simulink model "GPC"  (R2025b)
settings: Solver=FixedStepAuto  StartTime=0.0  StopTime=10.0  RelTol=1e-3
model workspace (MAT data in the model file):
  A = reshape([1 1 1 1 1 1 1 1 1 0.0375840959276 -0.0138679170576 -0.26090854365 0.179130502621 0.033894052833 0.0236937396522 0.00188563424393 -0.0137292088517 -0.225147986097 -0.282059074714 -0.0208812255081 0.110151665356 0.251260446677 -0.117899657826 -0.166134716199 -0.197559283491 -0.0255196194892 -0.044091775752 -0.336519979766 0.0187297142758 0.0478749224565 -0.137698933084 -0.35438494619 0.192962428222 0.00475946983706 0.0213883941121 -0.31920636287 -0.0980246146855 0.0103154407684 -0.0398902297506 0.0254465336583 -0.176213728897 -0.0657108585119 -0.0426588905364 0.00598757531626 -0.0347101416777 -0.0960427281846 0.0145828177398 -0.0190829804402 0.0914615693001 -0.160320038871 -0.147671747218 0.0154294464386 0.00151624371842 -0.102514250384], [3 3 6])
  B = reshape([0.00459780777595 1.42712475674e-05 -0.000408041445028 -0.00237157306223 0.00119304873837 0.000482775458328 0.00223132451004 0.000286686912328 0.00599135916028 0.0148665205586 5.139693558e-05 -0.00265500051912 -0.00735163394133 0.00391460700889 0.00243583441326 0.00755730776847 0.000748730221682 0.0148040671963 0.00740132665718 -0.000229008808218 -0.00369283887868 -0.00297542223091 0.00220653401484 0.00209157033751 0.00350399653917 -9.59277212105e-05 0.0030543274579 0.00490088499125 -0.000268745976113 -0.000437929455165 -0.00192593035877 0.00199079743513 0.000615437038067 0.000339606715612 -0.000260130070202 0.00641986430148 0.00188631931206 -6.20353133168e-05 -0.000608242812709 -0.00124764831245 0.000778872732744 0.00128937420791 0.000541054894972 5.56413892428e-05 0.000905590664489 0.000995289355196 -6.55613468166e-05 -0.000860934223846 -0.0004545573316 0.000285028917598 0.000527317246035 -0.000728392089223 -0.000148880686854 0.00124465963027], [3 3 6])
  N1 = 1
  N2 = 15
  Nu = 1
  alpha = 0.5
  lam = [0.2 0.08 0.5]
values from neighbouring files (symbols this model uses):
  Ts_ctrl = 0.1    [ctrlSys.sldd]
  u_b = 0.5864    [ctrlSys.sldd]
settings Model: DataDictionary=ctrlSys.sldd  Creator=LYG  LastModifiedBy=LYG

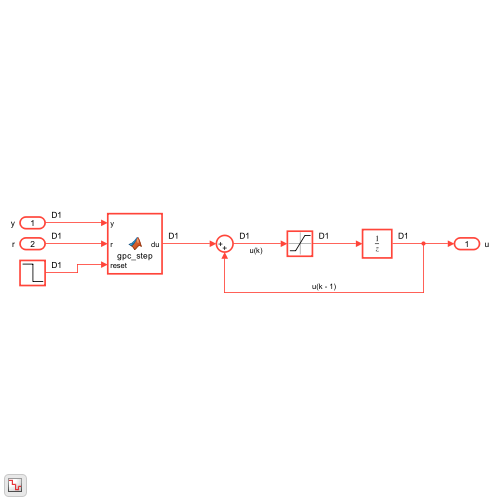
[thumbnail: Simulink's stored preview of the top-level diagram]
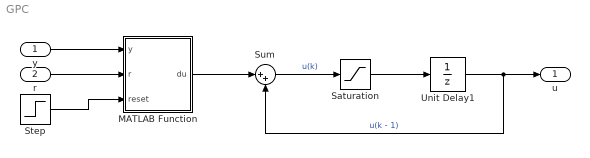
== system GPC ==
  y : Inport
  r : Inport  Port=2
  MATLAB Function : MATLAB Function  TreatAsAtomicUnit=on  SystemSampleTime=Ts_ctrl
  Saturation : Saturate  UpperLimit=1.12  LowerLimit=-1.08
  Step : Step  Time=0.5  Before=1  After=0  SampleTime=Ts_ctrl
  Sum : Sum  Inputs=|++
  Unit Delay1 : UnitDelay  InitialCondition=u_b  SampleTime=-1  HasFrameUpgradeWarning=on
  u : Outport
  wires:
  y/1 -> MATLAB Function/1(y)
  r/1 -> MATLAB Function/2(r)
  Saturation/1 -> Unit Delay1/1
  Sum/1 -> Saturation/1  "u(k)"
  MATLAB Function/1(du) -> Sum/1
  Unit Delay1/1 -> u/1, Sum/2  "u(k - 1)"
  Step/1 -> MATLAB Function/3(reset)

== matlab function GPC/MATLAB Function ==
  data: y input size=[3 1]; du output size=[3 1]; r input size=[3 1]; A parameter; B parameter; N1 parameter size=[1 1]; N2 parameter size=[1 1]; Nu parameter size=[1 1]; alpha parameter size=[1 1]; lam parameter size=[1 3]; reset input size=[1 1]
function du = gpc_step(y, r, A, B, N1, N2, Nu, alpha, lam, reset)
%GPC_STEP  One-step 3x3 GPC move for a CARIMA/ARIMA model with incremental control.
%   Codegen-friendly version for MATLAB Function blocks (no cell arrays).
%
%   A and B must be numeric arrays sized:
%     A: 3x3x(na+1) with A(:,:,1) == 1
%     B: 3x3x(nb+1)
%
%   Computes free response F and reference trajectory R, then applies
%   ΔU* = (G'G+λI)^{-1} G' (R-F) and outputs Δu(k) for each input.
%   Maintains histories of Δy and Δu between calls for the predictor.
    persistent K y_prev dy_hist du_hist last_A last_B last_N1 last_N2 last_Nu last_lam init_flag

    % Reset handling for MATLAB Function block.
    if isempty(init_flag)
        init_flag = true;
    end
    if reset
        init_flag = true;
        du = zeros(3, 1);
        return;
    end

    % Initialize cached parameters to avoid use-before-assign errors.
    if isempty(last_A)
        last_A = A;
        last_B = B;
        last_N1 = N1;
        last_N2 = N2;
        last_Nu = Nu;
        last_lam = lam;
    end

    % Cache the gain matrix unless model/horizons/weight change.
    if init_flag || isempty(K) || isempty(last_A) || isempty(last_B) || ...
            ~isequal(A, last_A) || ~isequal(B, last_B) || ...
            N1 ~= last_N1 || N2 ~= last_N2 || Nu ~= last_Nu || ~isequal(lam, last_lam)
        G = gmat(A, B, N1, N2, Nu);
        Lam = eye(3 * Nu);
        for i = 1:3
            r0 = (i - 1) * Nu + 1;
            Lam(r0:r0+Nu-1, r0:r0+Nu-1) = lam(i) * Lam(r0:r0+Nu-1, r0:r0+Nu-1);
        end
        K = (G' * G + Lam) \ G';
        last_A = A;
        last_B = B;
        last_N1 = N1;
        last_N2 = N2;
        last_Nu = Nu;
        last_lam = lam;
    end

    y = y(:);
    r = r(:);
    if numel(y) ~= 3 || numel(r) ~= 3
        error('y and r must be 3x1 vectors.');
    end

    if isscalar(alpha)
        alpha_vec = repmat(alpha, 3, 1);
    elseif numel(alpha) == 3
        alpha_vec = alpha(:);
    else
        error('alpha must be a scalar or a 3-element vector.');
    end

    % Initialize state history on first call.
    if init_flag || isempty(y_prev)
        y_prev = y;
    end
    na = size(A, 3) - 1;
    nb = size(B, 3) - 1;
    if init_flag || isempty(dy_hist)
        dy_hist = zeros(3, max(na, 1));
    end
    if init_flag || isempty(du_hist)
        du_hist = zeros(3, nb + 1);
    end
    init_flag = false;

    % Current output increment.
    dy_k = y - y_prev;

    % Build histories that include the current sample for free response.
    if na > 0
        dy_hist_use = [dy_k, dy_hist(:, 1:end-1)];
    else
        dy_hist_use = dy_hist(:, 1:1);
    end
    % Free response assumes Δu(k) = 0 (future moves handled by G*ΔU).
    du_hist_use = [zeros(3, 1), du_hist(:, 1:end-1)];

    % Free response over N1..N2.
    F = fmat(A, B, N1, N2, y, dy_hist_use, du_hist_use);

    % Reference trajectory over N1..N2 with exponential smoothing.
    Rfull = zeros(N2+1, 3);
    Rfull(1, :) = y.';
    for i = 2:N2+1
        alpha_row = alpha_vec.';
        Rfull(i, :) = alpha_row .* Rfull(i - 1, :) + (1 - alpha_row) .* r.';
    end
    rows = N2 - N1 + 1;
    R = zeros(3 * rows, 1);
    for i = 1:3
        r_i = Rfull(N1+1:N2+1, i);
        r0 = (i - 1) * rows + 1;
        R(r0:r0+rows-1) = r_i;
    end

    % Optimal move sequence and current move for each input.
    dU_star = K * (R - F);
    du = zeros(3, 1);
    du(1) = dU_star(1);
    du(2) = dU_star(Nu + 1);
    du(3) = dU_star(2 * Nu + 1);

    % Update histories for next call.
    du_hist = [du, du_hist(:, 1:end-1)];
    if na > 0
        dy_hist = [dy_k, dy_hist(:, 1:end-1)];
    end
    y_prev = y;
end
